simulink model "first_cl_dist_clean"  (R2021a)
settings: Solver=VariableStepAuto  StartTime=0.0  StopTime=5  RelTol=1e-3
values from neighbouring files (symbols this model uses):
  dist = [0;pi/(180/100);0;0]    [ex2main.m]
  K = lqr(sys,Q,R)    [ex2main.m]
  sys = get_fullstate_system(params)    [ex2main.m]
  x_d = desired_state(theta_d, params)    [ex2main.m]
settings Model: Creator=martijndebeuf  LastModifiedBy=martijndebeuf
settings SolverCC: AlgebraicLoopSolver=TrustRegion
settings DebuggingCC: SFMachineParentedDataDiag=warning

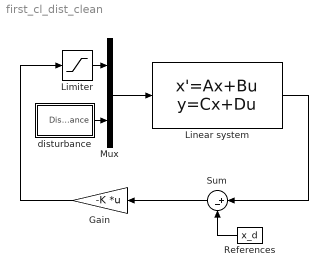
== system first_cl_dist_clean ==
  Gain : Gain  Gain=-K  Multiplication=Matrix(K*u) (u vector)
  Limiter : Saturate  UpperLimit=5  LowerLimit=-5
  Linear system : StateSpace  A=sys.A  B=[sys.B,dist]  C=sys.C  D=[sys.D,zeros(4,1)]  InitialCondition=initial_conditions'
  Mux : Mux  Inputs=2
  References : Constant  Value=x_d
  Sum : Sum  Inputs=|+-
  disturbance : Subsystem
  wires:
  Sum/1 -> Gain/1
  References/1 -> Sum/2
  Gain/1 -> Limiter/1
  Limiter/1 -> Mux/1
  Mux/1 -> Linear system/1
  Linear system/1 -> Sum/1
  disturbance/1(Disturbance) -> Mux/2

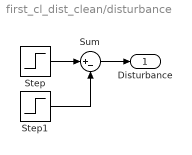
== system first_cl_dist_clean/disturbance ==
  Step : Step  SampleTime=0
  Step1 : Step  Time=1.1  SampleTime=0
  Sum : Sum  Inputs=|+-
  Disturbance : Outport
  wires:
  Sum/1 -> Disturbance/1
  Step1/1 -> Sum/2
  Step/1 -> Sum/1
